simulink model "quad_1_ref"  (R2018b)
settings: Solver=VariableStepAuto  StartTime=0.0  StopTime=options.T_train  RelTol=1e-3
undefined symbols (not defined in the file or in its folder): options
libraries: simulink x3
settings Model: Creator=kekatos  LastModifiedBy=kekatos

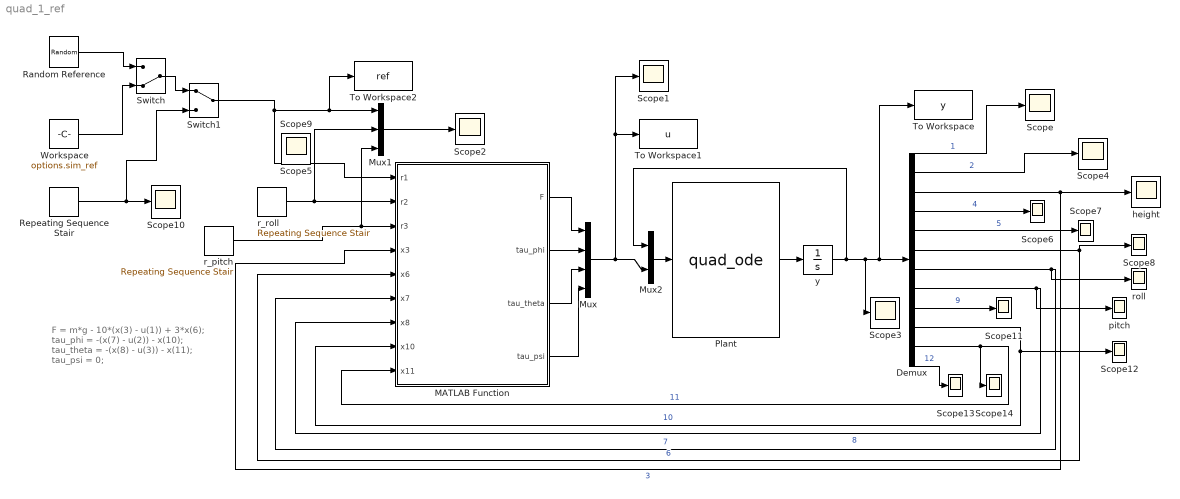
== system quad_1_ref ==
  note: F = m*g - 10*(x(3) - u(1)) + 3*x(6);
      |  tau_phi = -(x(7) - u(2)) - x(10);
      |  tau_theta = -(x(8) - u(3)) - x(11);
      | tau_psi = 0;
  Demux : Demux  Outputs=12
  MATLAB Function : MATLAB Function  TreatAsAtomicUnit=on
  Mux : Mux
  Mux1 : Mux  Inputs=3
  Mux2 : Mux  Inputs=2
  Plant : MATLABFcn  MATLABFcn=quad_ode  OutputDimensions=12
  Random Reference : UniformRandomNumber  Minimum=options.ref_min  Maximum=options.ref_max  Seed=randi(2^32,[1 ])  SampleTime=options.ref_Ts
  Repeating Sequence Stair : simulink/Sources/Repeating Sequence Stair  OutValues=options.sim_cov  tsamp=options.ref_Ts  OutMin=[]  OutMax=[]  OutDataTypeStr=double  OutputDataTypeScalingMode=double  OutDataType=fixdt(0,8)  ConRadixGroup=Best Precision: Vector-wise  OutScaling=2^-12
  Scope{,1..14} (15 alike) : Scope
  Switch : ManualSwitch  CurrentSetting=0
  Switch1 : ManualSwitch
  To Workspace : ToWorkspace  VariableName=y  SaveFormat=Structure With Time  SampleTime=0.01
  To Workspace1 : ToWorkspace  VariableName=u  SaveFormat=Structure With Time  SampleTime=0.01
  To Workspace2 : ToWorkspace  VariableName=ref  SaveFormat=Structure With Time  SampleTime=0.01
  Workspace : Constant  Value=options.sim_ref
  height : Scope
  pitch : Scope
  r_pitch : simulink/Sources/Repeating Sequence Stair  OutValues=0  tsamp=-1  OutMin=[]  OutMax=[]  OutDataTypeStr=double  OutputDataTypeScalingMode=double  OutDataType=fixdt(0,8)  ConRadixGroup=Best Precision: Vector-wise  OutScaling=2^-12
  r_roll : simulink/Sources/Repeating Sequence Stair  OutValues=0  tsamp=-1  OutMin=[]  OutMax=[]  OutDataTypeStr=double  OutputDataTypeScalingMode=double  OutDataType=fixdt(0,8)  ConRadixGroup=Best Precision: Vector-wise  OutScaling=2^-12
  roll : Scope
  y : Integrator  InitialCondition=options.simin_x0  ZeroCross=off
  wires:
  MATLAB Function/1(F) -> Mux/1
  MATLAB Function/2(tau_phi) -> Mux/2
  MATLAB Function/3(tau_theta) -> Mux/3
  MATLAB Function/4(tau_psi) -> Mux/4
  Switch1/1 -> MATLAB Function/1(r1), To Workspace2/1, Mux1/1
  r_roll/1 -> Mux1/2, MATLAB Function/2(r2)
  Demux/3 -> height/1, MATLAB Function/4(x3)  "3"
  Demux/6 -> Scope8/1, MATLAB Function/5(x6)  "6"
  Demux/7 -> roll/1, MATLAB Function/6(x7)  "7"
  Demux/8 -> pitch/1, MATLAB Function/7(x8)  "8"
  Demux/10 -> Scope12/1, MATLAB Function/8(x10)  "10"
  Demux/11 -> Scope14/1, MATLAB Function/9(x11)  "11"
  Demux/1 -> Scope/1  "1"
  Demux/2 -> Scope4/1  "2"
  Demux/4 -> Scope6/1  "4"
  Demux/5 -> Scope7/1  "5"
  Demux/9 -> Scope11/1  "9"
  Mux/1 -> Scope1/1, To Workspace1/1, Mux2/2
  Mux1/1 -> Scope2/1
  r_pitch/1 -> Mux1/3, MATLAB Function/3(r3)
  Demux/12 -> Scope13/1  "12"
  Plant/1 -> y/1
  Mux2/1 -> Plant/1
  y/1 -> Scope3/1, To Workspace/1, Demux/1, Mux2/1
  Random Reference/1 -> Switch/1
  Workspace/1 -> Switch/2
  Repeating Sequence Stair/1 -> Switch1/2, Scope10/1
  Switch/1 -> Switch1/1

== matlab function quad_1_ref/MATLAB Function ==
  data: r1 input; F output; r2 input; r3 input; x3 input; x6 input; x7 input; x8 input; x10 input; x11 input; tau_phi output; tau_theta output; tau_psi output
function [F,tau_phi,tau_theta,tau_psi] = fcn(r1,r2,r3,x3,x6,x7,x8,x10,x11)
%initialization
m=1.4;
g=9.81;
F= m*g-10*(x3-r1)+3*x6;
tau_phi=-(x7-r2)-x10;
tau_theta=-(x8-r3)-x11;
tau_psi=0;
